simulink model "test_PhaseSep_MeF"  (R2016a)
settings: Solver=ode15s  StartTime=0.0  StopTime=2e4  MaxStep=1e2  RelTol=1e-3
libraries: nesl_utility x20, simCryogenics_lib x18, fl_lib x4, simulink x2
settings Model: Creator=SK248285  LastModifiedBy=FB229602
settings DataIOCC: LimitDataPoints=on  SaveFormat=Array  SaveState=on
settings HardwareCC: ProdBitPerPointer=32  ProdLargestAtomicFloat=None  ProdIntDivRoundTo=Undefined  ProdEndianess=Unspecified  ProdWordSize=32  ProdHWDeviceType=32-bit Generic
settings ModelReferenceCC: PropagateSignalLabelsOutOfModel=off
settings ConfigComp: CovModelRefEnable=Off
settings SimscapeCC: SimscapeLogType=all  SimscapeLogLimitData=off

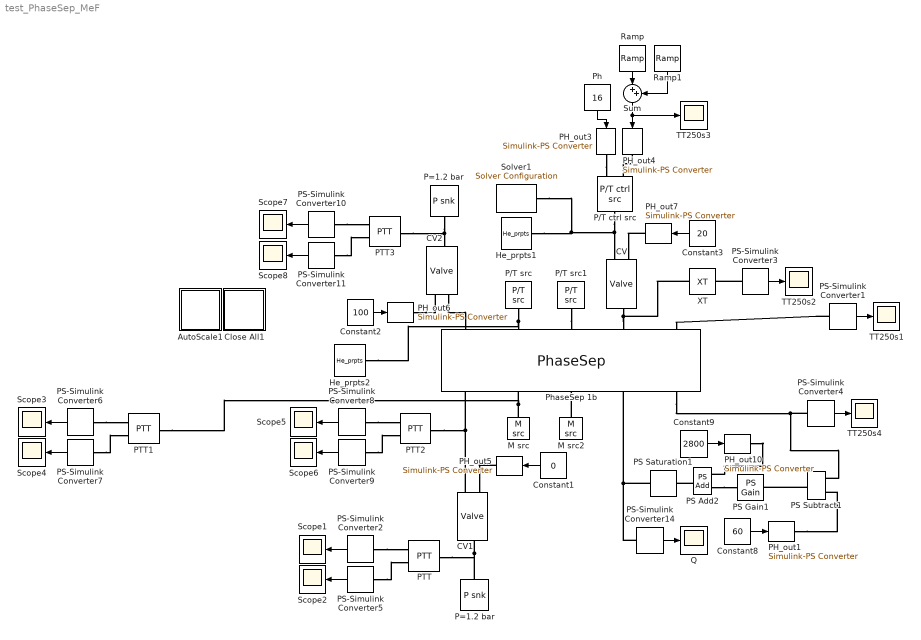
== system test_PhaseSep_MeF ==
  AutoScale1 : Subsystem
      settings: OpenFcn=|
      | set(0, 'showhiddenhandles', 'on')
      | 
      | scope = findobj(0, 'Tag', 'SIMULINK_SIMSCOPE_FIGURE');
      | 
      | for i=1:length(scope)
      |   simscope('ScopeBar', 'ActionIcon', 'Find',     scope(i))
      | end
      | 
      | set(0, 'showhiddenhandles', 'off')
      mask Display: disp('Auto\nScale\nScope')
  CV : simCryogenics_lib/Elements/Valve  CVmax=113  ControlInputMin=0  ControlInputMax=100  Xt=0.65  Rv=50  lin_v=0  lim_v=0  K=2.4e-5 m^1.50000*kg^0.50000/s/bar^0.50000  Cmd_specify=off  Cmd_priority=High  Cmd=0  gamma_specify=off  gamma_priority=High  gamma=0  rho_specify=off  rho_priority=High  rho=0 kg/m^3  Xc_specify=off  Xc_priority=High  Xc=0  X_specify=off  X_priority=High  X=0  Y_specify=off  Y_priority=High  Y=0  CV_specify=off  CV_priority=High  CV=0
  CV1 : simCryogenics_lib/Elements/Valve  CVmax=113  ControlInputMin=0  ControlInputMax=100  Xt=0.65  Rv=50  lin_v=0  lim_v=0  K=2.4e-5 m^1.50000*kg^0.50000/s/bar^0.50000  Cmd_specify=off  Cmd_priority=High  Cmd=0  gamma_specify=off  gamma_priority=High  gamma=0  rho_specify=off  rho_priority=High  rho=0 kg/m^3  Xc_specify=off  Xc_priority=High  Xc=0  X_specify=off  X_priority=High  X=0  Y_specify=off  Y_priority=High  Y=0  CV_specify=off  CV_priority=High  CV=0
  CV2 : simCryogenics_lib/Elements/Valve  CVmax=300  ControlInputMin=0  ControlInputMax=100  Xt=0.65  Rv=50  lin_v=0  lim_v=0  K=2.4e-5 m^1.50000*kg^0.50000/s/bar^0.50000  Cmd_specify=off  Cmd_priority=High  Cmd=0  gamma_specify=off  gamma_priority=High  gamma=0  rho_specify=off  rho_priority=High  rho=0 kg/m^3  Xc_specify=off  Xc_priority=High  Xc=0  X_specify=off  X_priority=High  X=0  Y_specify=off  Y_priority=High  Y=0  CV_specify=off  CV_priority=High  CV=0
  Close All1 : Subsystem
      settings: OpenFcn=|
      | set(0, 'showhiddenhandles', 'on')
      | scope = findobj(0, 'Tag','SIMULINK_SIMSCOPE_FIGURE');
      | close(scope)
      | set(0, 'showhiddenhandles', 'off')
      mask Display: disp('Close\nAll\nScope')
  Constant1 : Constant  Value=0
  Constant2 : Constant  Value=100
  Constant3 : Constant  Value=20
  Constant8 : Constant  Value=60
  Constant9 : Constant  Value=2800
  He_prpts1 : simCryogenics_lib/Utilities/He_prpts  P_min=1 bar  T_min=4 K  T_max=80 K  P_max=20 bar  Mol=4.0026 * 10 ^ (- 3) kg/mol
  He_prpts2 : simCryogenics_lib/Utilities/He_prpts  P_min=1 bar  T_min=4 K  T_max=80 K  P_max=20 bar  Mol=4.0026 * 10 ^ (- 3) kg/mol
  M src : simCryogenics_lib/Sources_Sinks/M src  M=0.01 kg/s
  M src2 : simCryogenics_lib/Sources_Sinks/M src  M=0 kg/s
  P/T ctrl src : simCryogenics_lib/Sources_Sinks/P//T ctrl src
  P/T src : simCryogenics_lib/Sources_Sinks/P//T src  P=1.1 bar  T=10 K
  P/T src1 : simCryogenics_lib/Sources_Sinks/P//T src  P=1.1 bar  T=10 K
  P=1.2 bar : simCryogenics_lib/Sources_Sinks/P snk  P=1.2 bar
  "P=1.2 bar " : simCryogenics_lib/Sources_Sinks/P snk  P=1.2 bar
  PH_out1 : nesl_utility/Simulink-PS Converter  PhysicalDomain=network_engine_domain  SubClassName=ps_input  LeftPortType=input  RightPortType=output  PseudoPeriodic=off  Frequencies=[]  NoiseDistribution=none  NoiseParameters=[]  Unit=bar  AffineConversion=off  InputFiltering=on  SimscapeFilterOrder=1  InputFilterTimeConstant=0.001  UdotUserProvided=1
  PH_out10 : nesl_utility/Simulink-PS Converter  PhysicalDomain=network_engine_domain  SubClassName=ps_input  LeftPortType=input  RightPortType=output  PseudoPeriodic=off  Frequencies=[]  NoiseDistribution=none  NoiseParameters=[]  Unit=bar  AffineConversion=off  InputFiltering=on  SimscapeFilterOrder=1  InputFilterTimeConstant=0.001  UdotUserProvided=1
  PH_out{3,5..7} (4 alike) : nesl_utility/Simulink-PS Converter  PhysicalDomain=network_engine_domain  SubClassName=ps_input  LeftPortType=input  RightPortType=output  PseudoPeriodic=off  Frequencies=[]  NoiseDistribution=none  NoiseParameters=[]  Unit=bar  AffineConversion=off  InputFiltering=off  SimscapeFilterOrder=1  InputFilterTimeConstant=0.001  UdotUserProvided=1
  PH_out4 : nesl_utility/Simulink-PS Converter  PhysicalDomain=network_engine_domain  SubClassName=ps_input  LeftPortType=input  RightPortType=output  PseudoPeriodic=off  Frequencies=[]  NoiseDistribution=none  NoiseParameters=[]  Unit=K  AffineConversion=off  InputFiltering=off  SimscapeFilterOrder=1  InputFilterTimeConstant=0.001  UdotUserProvided=1
  PS Add2 : fl_lib/Physical Signals/Functions/PS Add
  PS Gain1 : fl_lib/Physical Signals/Functions/PS Gain  gain=200
  PS Saturation1 : fl_lib/Physical Signals/Nonlinear Operators/PS Saturation  upper_limit=inf  lower_limit=-5
  PS Subtract1 : fl_lib/Physical Signals/Functions/PS Subtract
  PS-Simulink Converter{1..11,14} (12 alike) : nesl_utility/PS-Simulink Converter  PhysicalDomain=network_engine_domain  SubClassName=ps_output  LeftPortType=input  RightPortType=output  PseudoPeriodic=off  Frequencies=[]  Unit=1  AffineConversion=off
  PTT{,1..3} (4 alike) : simCryogenics_lib/Sensors/PTT
  Ph : Constant  Value=16
  PhaseSep 1b : simCryogenics_lib/Elements/PhaseSep  Ideal1=1  DeltaT1=0.05 K  N1=10  h1=950.3318 W/K  Ideal2=1  DeltaT2=0.05 K  N2=10  h2=950.3318 W/K  hmax=2.1 m  S=1 m^2  P0=1.2 bar  h0=0  T0=80 K
  Q : Scope
  Ramp : simulink/Sources/Ramp  slope=-75/(1e4)  start=0  X0=80
  Ramp1 : simulink/Sources/Ramp  slope=75/(1e4)  start=1e4  X0=0
  Scope{1..8} (8 alike) : Scope
  Solver1 : nesl_utility/Solver Configuration  PhysicalDomain=network_engine_domain  SubClassName=solver  LeftPortType=input  RightPortType=generic  Accelerate=off  Tones=[]  Harmonics=[]  SimulateNoise=off  Profile=off  UseLocalSampling=off  EnableSwitchedLinearOptims=on  FrequencyDomain=off  UseCCode=off  RelTol=0.001  AbsTol=1e-06  MinStep=1e-09  ToWorkspace=off  RevertToSquareIcSolve=off  NumHomotopyIterations=100  PhasorMode=off  PhasorModeNumHarmonics=1  OverrideAbsTol=off  DoDC=off  ResidualTolerance=1e-09  UseLocalSolver=off  LocalSolverChoice=NE_BACKWARD_EULER_ADVANCER  LocalSolverSampleTime=5  DoFixedCost=off  MaxNonlinIter=3  MaxModeIter=2  LinearAlgebra=Sparse  DelaysMemoryBudget=1024  AutomaticFiltering=on  FilteringTimeConstant=0.001
  Sum : Sum  Inputs=|++
  TT250s{1..4} (4 alike) : Scope
  XT : simCryogenics_lib/Sensors/XT
  wires:
  Sum/1 -> TT250s3/1, PH_out4/1
  Ph/1 -> PH_out3/1
  PS-Simulink Converter1/1 -> TT250s1/1
  Constant2/1 -> PH_out6/1
  Constant3/1 -> PH_out7/1
  Constant1/1 -> PH_out5/1
  PS-Simulink Converter2/1 -> Scope1/1
  PS-Simulink Converter5/1 -> Scope2/1
  PS-Simulink Converter8/1 -> Scope5/1
  PS-Simulink Converter9/1 -> Scope6/1
  PS-Simulink Converter10/1 -> Scope7/1
  PS-Simulink Converter11/1 -> Scope8/1
  PS-Simulink Converter3/1 -> TT250s2/1
  Constant8/1 -> PH_out1/1
  Constant9/1 -> PH_out10/1
  PS-Simulink Converter14/1 -> Q/1
  PS-Simulink Converter4/1 -> TT250s4/1
  PS-Simulink Converter6/1 -> Scope3/1
  PS-Simulink Converter7/1 -> Scope4/1
  Ramp/1 -> Sum/1
  Ramp1/1 -> Sum/2
  connections:
  PH_out3/RConn1 -- P/T ctrl src/LConn1
  P/T ctrl src/LConn2 -- PH_out4/RConn1
  He_prpts1/RConn1 -- Solver1/RConn1 -- CV/LConn2 -- P/T ctrl src/RConn1
  M src/RConn1 -- PTT1/LConn1 -- PhaseSep 1b/RConn2
  CV1/LConn2 -- PTT2/LConn1 -- PhaseSep 1b/RConn1
  CV2/LConn2 -- PhaseSep 1b/LConn1
  P/T src/RConn1 -- PhaseSep 1b/LConn2 -- He_prpts2/RConn1
  M src2/RConn1 -- PhaseSep 1b/RConn3
  PS-Simulink Converter1/LConn1 -- PhaseSep 1b/LConn5
  CV/RConn1 -- XT/LConn1 -- PhaseSep 1b/LConn4
  P/T src1/RConn1 -- PhaseSep 1b/LConn3
  PH_out6/RConn1 -- CV2/LConn1
  PH_out7/RConn1 -- CV/LConn1
  PH_out5/RConn1 -- CV1/LConn1
  P=1.2 bar/RConn1 -- PTT3/LConn1 -- CV2/RConn1
  CV1/RConn1 -- "P=1.2 bar "/RConn1 -- PTT/LConn1
  PhaseSep 1b/RConn5 -- PS Subtract1/LConn1 -- PS-Simulink Converter4/LConn1
  PS-Simulink Converter2/LConn1 -- PTT/RConn1
  PS-Simulink Converter5/LConn1 -- PTT/RConn2
  PS-Simulink Converter9/LConn1 -- PTT2/RConn2
  PS-Simulink Converter8/LConn1 -- PTT2/RConn1
  PS-Simulink Converter10/LConn1 -- PTT3/RConn1
  PS-Simulink Converter11/LConn1 -- PTT3/RConn2
  PS Saturation1/RConn1 -- PhaseSep 1b/RConn4 -- PS-Simulink Converter14/LConn1
  PS-Simulink Converter3/LConn1 -- XT/RConn1
  PS Add2/RConn1 -- PS Saturation1/LConn1
  PS Add2/LConn2 -- PS Gain1/RConn1
  PH_out10/RConn1 -- PS Add2/LConn1
  PH_out1/RConn1 -- PS Subtract1/LConn2
  PS Subtract1/RConn1 -- PS Gain1/LConn1
  PS-Simulink Converter7/LConn1 -- PTT1/RConn2
  PS-Simulink Converter6/LConn1 -- PTT1/RConn1

== system test_PhaseSep_MeF/AutoScale1 ==

== system test_PhaseSep_MeF/Close All1 ==
